simulink model "playback_data_4"  (R2015a)
settings: Solver=FixedStepDiscrete  SolverMode=SingleTasking  StartTime=0  StopTime=time_recorded(end)  FixedStep=sample_time  RelTol=1e-3
undefined symbols (not defined in the file): A1_notch_f1, A2_notch_f1, A_kalman_transverse, A_kalman_vertical, A_lpf_dtau, A_lpf_fourbar_angles, A_lpf_imu, A_lpf_lateral_angle, A_lpf_leg_spring, B1_lpf_dtau, B1_lpf_fourbar_angles, B1_lpf_imu, B1_lpf_lateral_angle, B1_lpf_leg_spring, B1_notch_f1, B2_lpf_dtau, B2_lpf_fourbar_angles, B2_lpf_imu, B2_lpf_lateral_angle, B2_lpf_leg_spring, B2_notch_f1, B_dx_versus_x0, B_kalman_transverse, B_kalman_vertical, backwards_K_front_of_t_row1, backwards_K_front_of_t_row2, backwards_K_sag_of_t, backwards_P_front_of_t, backwards_P_sag_of_t, C_kalman_transverse, C_kalman_vertical, com_leg_motor, com_torso, contact_threshold, control_start_time, d_ankle_to_foot, d_vertical_com, desired_com_forward_velocity, desired_com_lateral_velocity, desired_initial_leg_roll_left, desired_initial_leg_roll_right, desired_lateral_symmetry_angle, desired_standing_torso_pitch, desired_standing_torso_roll, desired_standing_z, desired_torso_pitch, desired_torso_roll, Discrete, fcut_contact, forward_dx_of_dxstar, forward_x_of_dxstar, g, gain_nodes_sea_torque, HIP_MTR_MAX_CONT_TORQUE, HIP_MTR_MAX_TORQUE, i_leg_motor, i_robot, i_torso, initial_dx_estimate, initial_dy_estimate ... (+75)
libraries: simulink x12, ctrlSharedLib x3
(part 2 of 5)

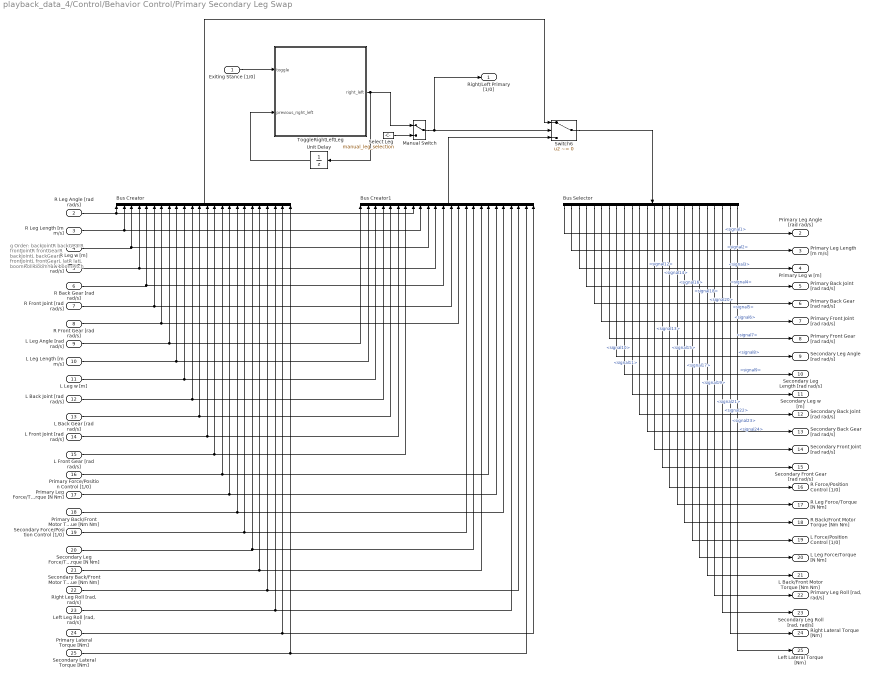
== system playback_data_4/Control/Behavior Control/Primary Secondary Leg Swap ==
  note: q Order:
      |
      | backJointR
      | backGearR
      | frontJointR
      | frontGearR
      |
      | backJointL
      | backGearL
      | frontJointL
      | frontGearL
      |
      | latR
      | latL
      |
      | boomRoll
      | boomYaw
      | boomPitch
  Exiting Stance [1/0] : Inport
  R Leg Angle [rad rad/s] : Inport  Port=2
  R Leg Length [m m/s] : Inport  Port=3
  R Leg w [m] : Inport  Port=4
  R Back Joint [rad rad/s] : Inport  Port=5
  R Back Gear [rad rad/s] : Inport  Port=6
  R Front Joint [rad rad/s] : Inport  Port=7
  R Front Gear [rad rad/s] : Inport  Port=8
  L Leg Angle [rad rad/s] : Inport  Port=9
  L Leg Length [m m/s] : Inport  Port=10
  L Leg w [m] : Inport  Port=11
  L Back Joint [rad rad/s] : Inport  Port=12
  L Back Gear [rad rad/s] : Inport  Port=13
  L Front Joint [rad rad/s] : Inport  Port=14
  L Front Gear [rad rad/s] : Inport  Port=15
  Primary Force/Position Control [1/0] : Inport  Port=16
  Primary Leg Force/Torque [N Nm] : Inport  Port=17
  Primary Back/Front Motor Torque [Nm Nm] : Inport  Port=18
  Secondary Force/Position Control [1/0] : Inport  Port=19
  Secondary Leg Force/Torque [N Nm] : Inport  Port=20
  Secondary Back/Front Motor Torque [Nm Nm] : Inport  Port=21
  "Right Leg Roll [rad, rad/s]" : Inport  Port=22
  "Left Leg Roll [rad, rad/s]" : Inport  Port=23
  Primary Lateral Torque [Nm] : Inport  Port=24
  Secondary Lateral Torque [Nm] : Inport  Port=25
  Bus Creator : BusCreator  Inputs=24
  Bus Creator1 : BusCreator  Inputs=24
  Bus Selector : BusSelector  OutputSignals=signal1,signal2,signal3,signal4,signal5,signal6,signal7,signal8,signal9,signal10,signal11,signal12,signal13,signal14,signal15,signal16,signal17,signal18,signal19,signal20,signal21,signal22,signal23,signal24
  Manual Switch : ManualSwitch
  Select Leg : Constant  Value=manual_leg_selection  OutDataTypeStr=boolean
  Switch6 : Switch  Criteria=u2 ~= 0  OutDataTypeStr=Inherit: Inherit via back propagation  ZeroCross=off
  ToggleRightLeftLeg : MATLAB Function  TreatAsAtomicUnit=on
      settings: MinAlgLoopOccurrences=on
  Unit Delay : UnitDelay  InitialCondition=manual_leg_selection  SampleTime=sample_time
  Right/Left Primary [1/0] : Outport
  Primary Leg Angle [rad rad/s] : Outport  Port=2
  Primary Leg Length [m m/s] : Outport  Port=3
  Primary Leg w [m] : Outport  Port=4
  Primary Back Joint [rad rad/s] : Outport  Port=5
  Primary Back Gear [rad rad/s] : Outport  Port=6
  Primary Front Joint [rad rad/s] : Outport  Port=7
  Primary Front Gear [rad rad/s] : Outport  Port=8
  Secondary Leg Angle [rad rad/s] : Outport  Port=9
  Secondary Leg Length [rad rad/s] : Outport  Port=10
  Secondary Leg w [m] : Outport  Port=11
  Secondary Back Joint [rad rad/s] : Outport  Port=12
  Secondary Back Gear [rad rad/s] : Outport  Port=13
  Secondary Front Joint [rad rad/s] : Outport  Port=14
  Secondary Front Gear [rad rad/s] : Outport  Port=15
  R Force/Position Control [1/0] : Outport  Port=16
  R Leg Force/Torque [N Nm] : Outport  Port=17
  R Back/Front Motor Torque [Nm Nm] : Outport  Port=18
  L Force/Position Control [1/0] : Outport  Port=19
  L Leg Force/Torque [N Nm] : Outport  Port=20
  L Back/Front Motor Torque [Nm Nm] : Outport  Port=21
  "Primary Leg Roll [rad, rad/s]" : Outport  Port=22
  "Secondary Leg Roll [rad, rad/s]" : Outport  Port=23
  Right Lateral Torque [Nm] : Outport  Port=24
  Left Lateral Torque [Nm] : Outport  Port=25
  wires:
  Bus Selector/24 -> Left Lateral Torque [Nm]/1  "<signal24>"
  Bus Selector/23 -> Right Lateral Torque [Nm]/1  "<signal23>"
  Secondary Lateral Torque [Nm]/1 -> Bus Creator/24, Bus Creator1/23
  Primary Lateral Torque [Nm]/1 -> Bus Creator/23, Bus Creator1/24
  Bus Selector/22 -> "Secondary Leg Roll [rad, rad/s]"/1  "<signal22>"
  Bus Selector/21 -> "Primary Leg Roll [rad, rad/s]"/1  "<signal21>"
  "Left Leg Roll [rad, rad/s]"/1 -> Bus Creator/22, Bus Creator1/21
  "Right Leg Roll [rad, rad/s]"/1 -> Bus Creator/21, Bus Creator1/22
  Bus Selector/20 -> L Back/Front Motor Torque [Nm Nm]/1  "<signal20>"
  Bus Selector/19 -> L Leg Force/Torque [N Nm]/1  "<signal19>"
  Bus Selector/18 -> L Force/Position Control [1/0]/1  "<signal18>"
  Bus Selector/17 -> R Back/Front Motor Torque [Nm Nm]/1  "<signal17>"
  Bus Selector/16 -> R Leg Force/Torque [N Nm]/1  "<signal16>"
  Bus Selector/15 -> R Force/Position Control [1/0]/1  "<signal15>"
  Bus Selector/14 -> Secondary Front Gear [rad rad/s]/1  "<signal14>"
  Bus Selector/13 -> Secondary Front Joint [rad rad/s]/1  "<signal13>"
  Bus Selector/12 -> Secondary Back Gear [rad rad/s]/1  "<signal12>"
  Bus Selector/11 -> Secondary Back Joint [rad rad/s]/1  "<signal11>"
  Bus Selector/10 -> Secondary Leg w [m]/1  "<signal10>"
  Bus Selector/9 -> Secondary Leg Length [rad rad/s]/1  "<signal9>"
  Bus Selector/8 -> Secondary Leg Angle [rad rad/s]/1  "<signal8>"
  Bus Selector/7 -> Primary Front Gear [rad rad/s]/1  "<signal7>"
  Bus Selector/6 -> Primary Front Joint [rad rad/s]/1  "<signal6>"
  Bus Selector/5 -> Primary Back Gear [rad rad/s]/1  "<signal5>"
  Bus Selector/4 -> Primary Back Joint [rad rad/s]/1  "<signal4>"
  Bus Selector/3 -> Primary Leg w [m]/1  "<signal3>"
  Bus Selector/2 -> Primary Leg Length [m m/s]/1  "<signal2>"
  Bus Selector/1 -> Primary Leg Angle [rad rad/s]/1  "<signal1>"
  Switch6/1 -> Bus Selector/1
  Secondary Back/Front Motor Torque [Nm Nm]/1 -> Bus Creator/20, Bus Creator1/17
  Secondary Leg Force/Torque [N Nm]/1 -> Bus Creator/19, Bus Creator1/16
  Secondary Force/Position Control [1/0]/1 -> Bus Creator/18, Bus Creator1/15
  Primary Back/Front Motor Torque [Nm Nm]/1 -> Bus Creator/17, Bus Creator1/20
  Primary Leg Force/Torque [N Nm]/1 -> Bus Creator/16, Bus Creator1/19
  Primary Force/Position Control [1/0]/1 -> Bus Creator/15, Bus Creator1/18
  L Front Gear [rad rad/s]/1 -> Bus Creator/14, Bus Creator1/7
  L Front Joint [rad rad/s]/1 -> Bus Creator1/6, Bus Creator/13
  L Back Gear [rad rad/s]/1 -> Bus Creator/12, Bus Creator1/5
  L Back Joint [rad rad/s]/1 -> Bus Creator/11, Bus Creator1/4
  L Leg w [m]/1 -> Bus Creator/10, Bus Creator1/3
  L Leg Length [m m/s]/1 -> Bus Creator/9, Bus Creator1/2
  L Leg Angle [rad rad/s]/1 -> Bus Creator/8, Bus Creator1/1
  R Front Gear [rad rad/s]/1 -> Bus Creator/7, Bus Creator1/14
  R Front Joint [rad rad/s]/1 -> Bus Creator/6, Bus Creator1/13
  R Back Gear [rad rad/s]/1 -> Bus Creator/5, Bus Creator1/12
  R Back Joint [rad rad/s]/1 -> Bus Creator/4, Bus Creator1/11
  Bus Creator1/1 -> Switch6/3
  Bus Creator/1 -> Switch6/1
  R Leg Length [m m/s]/1 -> Bus Creator/2, Bus Creator1/9
  R Leg Angle [rad rad/s]/1 -> Bus Creator/1, Bus Creator1/8
  R Leg w [m]/1 -> Bus Creator/3, Bus Creator1/10
  Select Leg/1 -> Manual Switch/2
  Manual Switch/1 -> Switch6/2, Right/Left Primary [1/0]/1
  ToggleRightLeftLeg/1(right_left) -> Manual Switch/1, Unit Delay/1
  Exiting Stance [1/0]/1 -> ToggleRightLeftLeg/1(toggle)
  Unit Delay/1 -> ToggleRightLeftLeg/2(previous_right_left)

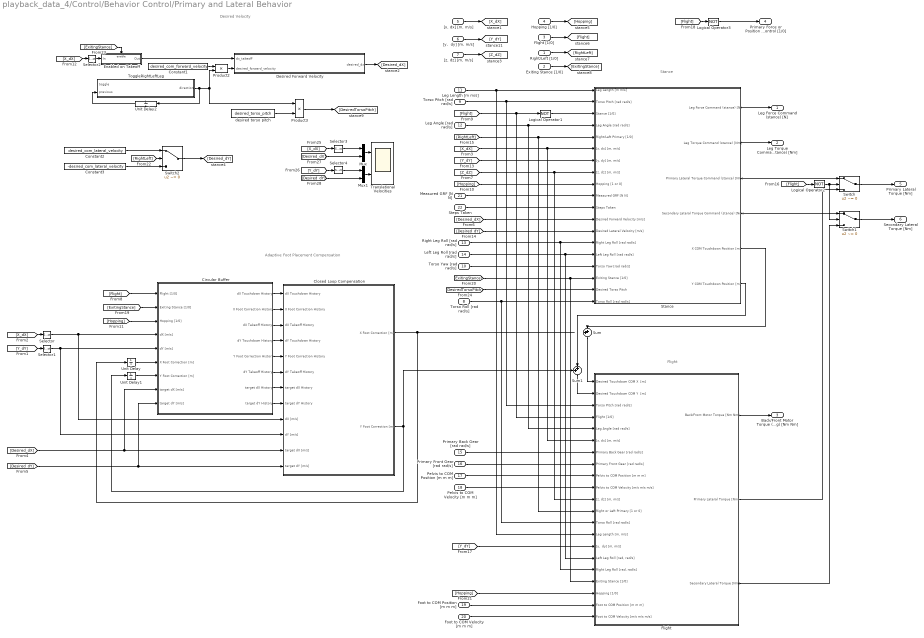
== system playback_data_4/Control/Behavior Control/Primary and Lateral Behavior ==
  note: Desired Velocity
  note: Adaptive Foot Placement Compensation
  note: Flight
  note: Stance
  Right/Left [1/0] : Inport
  Exiting Stance [1/0] : Inport  Port=2
  Flight [1/0] : Inport  Port=3
  Hopping [1/0] : Inport  Port=4
  "[x, dx] [m, m/s]" : Inport  Port=5
  "[y,  dy] [m, m/s]" : Inport  Port=6
  "[z, dz] [m, m/s]" : Inport  Port=7
  Torso Roll [rad rad/s] : Inport  Port=8
  Torso Pitch [rad rad/s] : Inport  Port=9
  Torso Yaw [rad rad/s] : Inport  Port=10
  Leg Length [m m/s] : Inport  Port=11
  Leg Angle [rad rad/s] : Inport  Port=12
  Right Leg Roll [rad rad/s] : Inport  Port=13
  Left Leg Roll [rad rad/s] : Inport  Port=14
  Primary Back Gear [rad rad/s] : Inport  Port=15
  Primary Front Gear [rad rad/s] : Inport  Port=16
  Pelvis to COM Position [m m m] : Inport  Port=17
  Pelvis to COM Velocity [m m m] : Inport  Port=18
  Foot to COM Position [m m m] : Inport  Port=19
  Foot to COM Velocity [m m m] : Inport  Port=20
  Measured GRF [N N] : Inport  Port=21
  Steps Taken : Inport  Port=22
  Circular Buffer : Subsystem
  Closed Loop Compensation : Subsystem
  Constant1 : Constant  Value=desired_com_forward_velocity
  Constant2 : Constant  Value=desired_com_lateral_velocity
  Constant3 : Constant  Value=-desired_com_lateral_velocity
  Desired Forward Velocity : MATLAB Function  TreatAsAtomicUnit=on
  Enabled on Takeoff : Subsystem  TreatAsAtomicUnit=on
  Flight : Subsystem
  Logical Operator1 : Logic  Operator=NOT  AllPortsSameDT=off  OutDataTypeStr=boolean
  Logical Operator2 : Logic  Operator=NOT  AllPortsSameDT=off  OutDataTypeStr=boolean
  Logical Operator3 : Logic  Operator=NOT  AllPortsSameDT=off  OutDataTypeStr=boolean
  Mux : Mux  Inputs=2
  Mux1 : Mux  Inputs=2
  Product2 : Product
  Product3 : Product
  Selector{,1..4} (5 alike) : Selector  InputPortWidth=2  Indices=[2]
  Stance : Subsystem
  Sum : Sum  Inputs=++|
  Sum1 : Sum  Inputs=++|
  Switch : Switch  Criteria=u2 ~= 0
  Switch1 : Switch  Criteria=u2 ~= 0
  Switch2 : Switch  Criteria=u2 ~= 0
  ToggleRightLeftLeg : MATLAB Function  TreatAsAtomicUnit=on
      settings: MinAlgLoopOccurrences=on
  Translational Velocities : Scope  NumInputPorts=2
      settings: YMin=-1000~-5  YMax=1000~5  SaveName=ScopeData2  SampleInput=on
  Unit Delay : UnitDelay  SampleTime=-1
  Unit Delay1 : UnitDelay  SampleTime=-1
  Unit Delay2 : UnitDelay  InitialCondition=1  SampleTime=sample_time
  desired torso pitch : Constant  Value=desired_torso_pitch
  Leg Force Command (stance) [N] : Outport
  Leg Torque Command (stance) [Nm] : Outport  Port=2
  Back/Front Motor Torque (swing) [Nm Nm] : Outport  Port=3
  Primary Force or Position Control [1/0] : Outport  Port=4  OutDataTypeStr=boolean
  Primary Lateral Torque [Nm] : Outport  Port=5
  Secondary Lateral Torque [Nm] : Outport  Port=6
  wires:
  [Desired_dX] -> Mux/2
  [Desired_dY] -> Mux1/2
  Mux1/1 -> Translational Velocities/2
  Mux/1 -> Translational Velocities/1
  Selector4/1 -> Mux1/1
  [Y_dY] -> Selector4/1
  Selector3/1 -> Mux/1
  [X_dX] -> Selector3/1
  Foot to COM Velocity [m m m]/1 -> Flight/21(Foot to COM Velocity [m/s m/s m/s])
  Foot to COM Position [m m m]/1 -> Flight/20(Foot to COM Position [m m m])
  [DesiredTorsoPitch] -> Stance/18(Desired Torso Pitch)
  Product3/1 -> [DesiredTorsoPitch]
  desired torso pitch/1 -> Product3/2
  Constant1/1 -> Product2/1
  Unit Delay2/1 -> ToggleRightLeftLeg/2(previous)
  ToggleRightLeftLeg/1(direction) -> Unit Delay2/1, Product3/1, Product2/2
  Product2/1 -> Desired Forward Velocity/2(desired_forward_velocity)
  Desired Forward Velocity/1(desired_dx) -> [Desired_dX]
  Selector2/1 -> Enabled on Takeoff/1(In)
  [ExitingStance] -> Enabled on Takeoff/Enable
  Constant3/1 -> Switch2/3
  Constant2/1 -> Switch2/1
  [RightLeft] -> Switch2/2
  Enabled on Takeoff/1(Out) -> Desired Forward Velocity/1(dx_takeoff)
  Switch2/1 -> [Desired_dY]
  [X_dX] -> Selector2/1
  [Hopping] -> Flight/19(Hopping [1/0])
  [ExitingStance] -> Flight/18(Exiting Stance [1/0]), Stance/17(Exiting Stance [1/0])
  Exiting Stance [1/0]/1 -> [ExitingStance]
  [ExitingStance] -> Circular Buffer/2(Exiting Stance [1/0])
  [Hopping] -> Circular Buffer/3(Hopping [1/0])
  Torso Yaw [rad rad/s]/1 -> Stance/16(Torso Yaw [rad rad/s])
  Logical Operator3/1 -> Primary Force or Position Control [1/0]/1
  [Flight] -> Logical Operator3/1
  Switch1/1 -> Secondary Lateral Torque [Nm]/1
  Switch/1 -> Primary Lateral Torque [Nm]/1
  [Flight] -> Logical Operator2/1
  Flight/3(Secondary Lateral Torque [Nm]) -> Switch1/3
  Stance/4(Secondary Lateral Torque Command (stance) [Nm]) -> Switch1/1
  Flight/2(Primary Lateral Torque [Nm]) -> Switch/3
  Stance/3(Primary Lateral Torque Command (stance) [Nm]) -> Switch/1
  Logical Operator2/1 -> Switch/2, Switch1/2
  Right/Left [1/0]/1 -> [RightLeft]
  [Desired_dY] -> Stance/13(Desired Lateral Velocity [m/s])
  [Y_dY] -> Stance/7("[y, dy] [m, m/s]")
  Left Leg Roll [rad rad/s]/1 -> Flight/16("Left Leg Roll [rad, rad/s]"), Stance/15(Left Leg Roll [rad rad/s])
  Right Leg Roll [rad rad/s]/1 -> Flight/17("Right Leg Roll [rad, rad/s]"), Stance/14(Right Leg Roll [rad rad/s])
  Sum1/1 -> Flight/2(Desired Touchdown COM Y  [m])
  Stance/6(Y COM Touchdown Position [m]) -> Sum1/2
  Hopping [1/0]/1 -> [Hopping]
  [Flight] -> Logical Operator1/1, Flight/4(Flight [1/0])
  Flight [1/0]/1 -> [Flight]
  [Desired_dX] -> Stance/12(Desired Forward Velocity [m/s])
  [Y_dY] -> Selector1/1
  [X_dX] -> Selector/1
  "[y,  dy] [m, m/s]"/1 -> [Y_dY]
  "[z, dz] [m, m/s]"/1 -> [Z_dZ]
  "[x, dx] [m, m/s]"/1 -> [X_dX]
  Closed Loop Compensation/2(Y Foot Correction [m]) -> Sum1/1, Unit Delay1/1
  Unit Delay/1 -> Circular Buffer/6(X Foot Correction [m])
  Unit Delay1/1 -> Circular Buffer/7(Y Foot Correction [m])
  Selector/1 -> Circular Buffer/4(dX [m/s]), Closed Loop Compensation/9(dX [m/s])
  Selector1/1 -> Circular Buffer/5(dY [m/s]), Closed Loop Compensation/10(dY [m/s])
  Closed Loop Compensation/1(X Foot Correction [m]) -> Unit Delay/1
  Sum/1 -> Flight/1(Desired Touchdown COM X  [m])
  Stance/5(X COM Touchdown Position [m]) -> Sum/2
  [Desired_dY] -> Closed Loop Compensation/12("target dY [m/s] "), Circular Buffer/9(target dY [m/s])
  [Desired_dX] -> Closed Loop Compensation/11(target dX [m/s]), Circular Buffer/8(target dX [m/s])
  Circular Buffer/7(target dX History) -> Closed Loop Compensation/7(target dX History)
  Circular Buffer/8(target dY History) -> Closed Loop Compensation/8(target dY History)
  Circular Buffer/6(dY Takeoff History) -> Closed Loop Compensation/6(dY Takeoff History)
  Circular Buffer/5(Y Foot Correction History) -> Closed Loop Compensation/5(Y Foot Correction History)
  Circular Buffer/4("dY Touchdown History ") -> Closed Loop Compensation/4(dY Touchdown History)
  Circular Buffer/3(dX Takeoff History) -> Closed Loop Compensation/3(dX Takeoff History)
  Circular Buffer/2(X Foot Correction History) -> Closed Loop Compensation/2(X Foot Correction History)
  Circular Buffer/1("dX Touchdown History ") -> Closed Loop Compensation/1(dX Touchdown History)
  [Y_dY] -> Flight/15("[y,  dy] [m, m/s]")
  Steps Taken/1 -> Stance/11(Steps Taken)
  Measured GRF [N N]/1 -> Stance/10(Measured GRF [N N])
  Torso Roll [rad rad/s]/1 -> Flight/13(Torso Roll [rad rad/s]), Stance/19(Torso Roll [rad rad/s])
  Pelvis to COM Velocity [m m m]/1 -> Flight/10(Pelvis to COM Velocity [m/s m/s m/s])
  [Z_dZ] -> Flight/11("[z, dz] [m, m/s]"), Stance/8("[z, dz] [m, m/s]")
  Pelvis to COM Position [m m m]/1 -> Flight/9(Pelvis to COM Position [m m m])
  [Flight] -> Circular Buffer/1(Flight [1/0])
  Logical Operator1/1 -> Stance/3(Stance [1/0])
  Flight/1(Back/Front Motor Torque [Nm Nm]) -> Back/Front Motor Torque (swing) [Nm Nm]/1
  Leg Angle [rad rad/s]/1 -> Flight/5(Leg Angle [rad rad/s]), Stance/4(Leg Angle [rad rad/s])
  Primary Front Gear [rad rad/s]/1 -> Flight/8(Primary Front Gear [rad rad/s])
  Primary Back Gear [rad rad/s]/1 -> Flight/7(Primary Back Gear [rad rad/s])
  [RightLeft] -> Flight/12(Right or Left Primary [1 or 0]), Stance/5(Right/Left Primary [1/0])
  [X_dX] -> Flight/6("[x, dx] [m, m/s]"), Stance/6("[x, dx] [m, m/s]")
  [Hopping] -> Stance/9(Hopping [1 or 0])
  Torso Pitch [rad rad/s]/1 -> Flight/3(Torso Pitch [rad rad/s]), Stance/2(Torso Pitch [rad rad/s])
  Stance/2(Leg Torque Command (stance) [Nm]) -> Leg Torque Command (stance) [Nm]/1
  Stance/1(Leg Force Command (stance) [N]) -> Leg Force Command (stance) [N]/1
  Leg Length [m m/s]/1 -> Flight/14("Leg Length [m, m/s]"), Stance/1(Leg Length [m m/s])

== system playback_data_4/Control/Behavior Control/R Leg Calculator ==
  Front [rad rad/s] : Inport
  Back [rad rad/s] : Inport  Port=2
  Constant : Constant  Value=d_ankle_to_foot-0.01
  Demux1 : Demux  Outputs=2
  Gain1 : Gain  Gain=2*l_seg
  Gain2 : Gain  Gain=l_seg
  Gain3 : Gain  Gain=-1
  Gain4 : Gain  Gain=0.5
  Gain5 : Gain  Gain=0.5
  Gain6 : Gain  Gain=2
  Mux1 : Mux  Inputs=2
  Product : Product  RndMeth=Zero
  Sum : Sum  Inputs=++|
  Sum4 : Sum  Inputs=+|+
  Sum5 : Sum  Inputs=+|-
  Trigonometric Function : Trigonometry  Operator=cos
  Trigonometric Function1 : Trigonometry
  "Leg Length [m m/s] " : Outport
  Leg Angle [rad rad/s] : Outport  Port=2
  Leg Splay [rad rad/s] : Outport  Port=3
  w [m] : Outport  Port=4
  wires:
  Gain5/1 -> Leg Angle [rad rad/s]/1
  Sum4/1 -> Gain5/1
  Mux1/1 -> "Leg Length [m m/s] "/1
  Sum5/1 -> Demux1/1, Leg Splay [rad rad/s]/1
  Gain2/1 -> Gain6/1, Product/1
  Demux1/1 -> Gain4/1
  Gain3/1 -> Product/2
  Demux1/2 -> Gain3/1
  Back [rad rad/s]/1 -> Sum5/1, Sum4/1
  Front [rad rad/s]/1 -> Sum4/2, Sum5/2
  Product/1 -> Mux1/2
  Trigonometric Function1/1 -> Gain2/1
  Gain1/1 -> Sum/2
  Trigonometric Function/1 -> Gain1/1
  Gain4/1 -> Trigonometric Function/1, Trigonometric Function1/1
  Gain6/1 -> w [m]/1
  Sum/1 -> Mux1/1
  Constant/1 -> Sum/1

== system playback_data_4/Control/Behavior Control/Secondary Leg Behavior ==
  note: Convert to
      | four-bar angles
  note: Position control the
      | individual four bar segments
  note: Mirror the primary
      | leg motion
  Secondary Back Gear [rad rad/s] : Inport
  Secondary Front Gear [rad rad/s] : Inport  Port=2
  Torso Pitch [rad rad/s] : Inport  Port=3
  Right/Left Secondary [1/0] : Inport  Port=4
  Primary Leg Angle [rad rad/s] : Inport  Port=5
  Primary Leg Length [m m/s] : Inport  Port=6
  Avoid Hitting Mechanical Limits : MATLAB Function  TreatAsAtomicUnit=on
  Back/Front Motor PD : Subsystem
  Constant4 : Constant  Value=0
  Constant5 : Constant  Value=0  OutDataTypeStr=boolean
  Demux{1..3,5} (4 alike) : Demux  Outputs=2
  Demux6 : Demux  Outputs=6
  Fcn2 : Fcn  Expr=2*pi-u(1)
  Mirrored Leg Length Target : MATLAB Function  TreatAsAtomicUnit=on
  Mux{1..4,7,11} (6 alike) : Mux  Inputs=2
  Mux5 : Mux  Inputs=3
  Mux6 : Mux  Inputs=3
  Sum1 : Sum  Inputs=++|
  Virtual Leg to Four Bar : MATLAB Function  TreatAsAtomicUnit=on
  k_virtual6 : Gain  Gain=-1
  two_pole_filter : DiscreteTransferFcn  Numerator=[A_lpf_leg_spring 0 0]  Denominator=[1 B1_lpf_leg_spring B2_lpf_leg_spring]  SampleTime=sample_time
  Secondary Back/Front Motor Torque [Nm Nm] : Outport
  Secondary Force or Position Control [1/0] : Outport  Port=2
  wires:
  Back/Front Motor PD/1(Commanded Torque [Nm] [back front]) -> Secondary Back/Front Motor Torque [Nm Nm]/1
  Primary Leg Length [m m/s]/1 -> Demux1/1
  Demux1/2 -> Mirrored Leg Length Target/2(primary_dl_leg)
  Demux1/1 -> Mirrored Leg Length Target/1(primary_l_leg)
  Sum1/1 -> Demux5/1
  two_pole_filter/1 -> Sum1/2
  Mux3/1 -> Back/Front Motor PD/3(Desired Acceleration [rad/s^2] [back front])
  Mux2/1 -> Back/Front Motor PD/2(Desired Velocity [rad/s] [back front])
  Avoid Hitting Mechanical Limits/6(ddfront_cmd) -> Mux3/2
  Avoid Hitting Mechanical Limits/5(ddback_cmd) -> Mux3/1
  Avoid Hitting Mechanical Limits/4(dfront_cmd) -> Mux2/2
  Avoid Hitting Mechanical Limits/3(dback_cmd) -> Mux2/1
  Secondary Back Gear [rad rad/s]/1 -> Demux3/1
  Secondary Front Gear [rad rad/s]/1 -> Demux2/1
  Demux2/1 -> Mux4/2
  Avoid Hitting Mechanical Limits/1(back_cmd) -> Mux1/1
  Avoid Hitting Mechanical Limits/2(front_cmd) -> Mux1/2
  Demux3/1 -> Mux4/1
  Demux3/2 -> Mux11/1
  Right/Left Secondary [1/0]/1 -> Back/Front Motor PD/6(Right/Left Leg [1/0])
  Mux1/1 -> Back/Front Motor PD/1(Desired Position [rad] [back front])
  Mux4/1 -> Back/Front Motor PD/4(Measured Position [rad] [back front])
  Demux2/2 -> Mux11/2
  Mux11/1 -> Back/Front Motor PD/5(Measured Velocity [rad/s] [back front])
  Demux6/6 -> Virtual Leg to Four Bar/6(ddphi)
  Demux6/5 -> Virtual Leg to Four Bar/5(dphi)
  Demux6/4 -> Virtual Leg to Four Bar/4(phi)
  Demux6/3 -> Virtual Leg to Four Bar/3(ddl_leg)
  Demux6/2 -> Virtual Leg to Four Bar/2(dl_leg)
  Demux6/1 -> Virtual Leg to Four Bar/1(l_leg)
  Virtual Leg to Four Bar/6(ddfront) -> Avoid Hitting Mechanical Limits/6(ddfront_desired)
  Virtual Leg to Four Bar/5(dfront) -> Avoid Hitting Mechanical Limits/5(dfront_desired)
  Virtual Leg to Four Bar/4(front) -> Avoid Hitting Mechanical Limits/4(front_desired)
  Virtual Leg to Four Bar/3(ddback) -> Avoid Hitting Mechanical Limits/3(ddback_desired)
  Virtual Leg to Four Bar/2(dback) -> Avoid Hitting Mechanical Limits/2(dback_desired)
  Virtual Leg to Four Bar/1(back) -> Avoid Hitting Mechanical Limits/1(back_desired)
  Mux6/1 -> Mux7/2
  Mux5/1 -> Mux7/1
  Torso Pitch [rad rad/s]/1 -> Sum1/1
  Mux7/1 -> Demux6/1
  Fcn2/1 -> Mux6/1
  k_virtual6/1 -> Mux6/2
  Constant4/1 -> Mux6/3
  Mirrored Leg Length Target/1(l_leg) -> Mux5/1
  Mirrored Leg Length Target/3(ddl_leg) -> Mux5/3
  Mirrored Leg Length Target/2(dl_leg) -> Mux5/2
  Primary Leg Angle [rad rad/s]/1 -> two_pole_filter/1
  Demux5/1 -> Fcn2/1
  Demux5/2 -> k_virtual6/1
  Constant5/1 -> Secondary Force or Position Control [1/0]/1

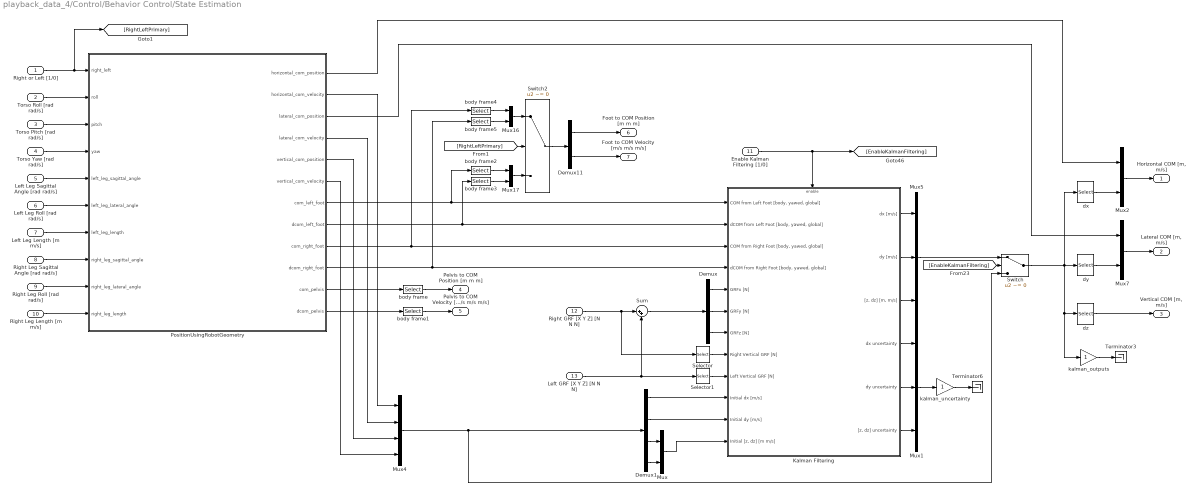
== system playback_data_4/Control/Behavior Control/State Estimation ==
  Right or Left [1/0] : Inport
  Torso Roll [rad rad/s] : Inport  Port=2
  Torso Pitch [rad rad/s] : Inport  Port=3
  Torso Yaw [rad rad/s] : Inport  Port=4
  Left Leg Sagittal Angle [rad rad/s] : Inport  Port=5
  Left Leg Roll [rad rad/s] : Inport  Port=6
  Left Leg Length [m m/s] : Inport  Port=7
  Right Leg Sagittal Angle [rad rad/s] : Inport  Port=8
  Right Leg Roll [rad rad/s] : Inport  Port=9
  Right Leg Length [m m/s] : Inport  Port=10
  Enable Kalman Filtering [1/0] : Inport  Port=11
  Right GRF [X Y Z] [N N N] : Inport  Port=12
  Left GRF [X Y Z] [N N N] : Inport  Port=13
  Demux : Demux  Outputs=3
  Demux1 : Demux
  Demux11 : Demux  Outputs=2
  Kalman Filtering : Subsystem
  Mux{,2,7,16..17} (5 alike) : Mux  Inputs=2
  Mux1 : Mux  Inputs=3
  Mux4 : Mux
  Mux5 : Mux  Inputs=3
  PositionUsingRobotGeometry : MATLAB Function  TreatAsAtomicUnit=on
  Selector : Selector  InputPortWidth=3  Indices=[3]
  Selector1 : Selector  InputPortWidth=3  Indices=[3]
  Sum : Sum  Inputs=|++
  Switch : Switch  Criteria=u2 ~= 0
  Switch2 : Switch  Criteria=u2 ~= 0
  Terminator3 : Terminator
  Terminator6 : Terminator
  body frame : Selector  InputPortWidth=9  Indices=[1 2 3]
  body frame1 : Selector  InputPortWidth=9  Indices=[1 2 3]
  body frame{2..5} (4 alike) : Selector  InputPortWidth=9  Indices=[4 5 6]
  dx : Selector  InputPortWidth=4  Indices=[1]
  dy : Selector  InputPortWidth=4  Indices=[2]
  dz : Selector  InputPortWidth=4  Indices=[3 4]
  kalman_outputs : Gain
  kalman_uncertainty : Gain
  "Horizontal COM [m, m/s]" : Outport
  "Lateral COM [m, m/s]" : Outport  Port=2
  "Vertical COM [m, m/s]" : Outport  Port=3
  Pelvis to COM Position [m m m] : Outport  Port=4
  Pelvis to COM Velocity [m/s m/s m/s] : Outport  Port=5
  Foot to COM Position [m m m] : Outport  Port=6
  Foot to COM Velocity [m/s m/s m/s] : Outport  Port=7
  wires:
  body frame4/1 -> Mux16/1
  body frame5/1 -> Mux16/2
  body frame3/1 -> Mux17/2
  body frame2/1 -> Mux17/1
  Demux11/1 -> Foot to COM Position [m m m]/1
  Demux11/2 -> Foot to COM Velocity [m/s m/s m/s]/1
  Switch2/1 -> Demux11/1
  Mux16/1 -> Switch2/1
  Mux17/1 -> Switch2/3
  [RightLeftPrimary] -> Switch2/2
  Demux1/1 -> Kalman Filtering/10(Initial dx [m/s])
  Demux1/2 -> Kalman Filtering/11(Initial dy [m/s])
  Mux/1 -> Kalman Filtering/12("Initial [z, dz] [m m/s]")
  Demux1/4 -> Mux/2
  Demux1/3 -> Mux/1
  Mux4/1 -> Switch/3, Demux1/1
  [EnableKalmanFiltering] -> Switch/2
  dy/1 -> Mux7/2
  Mux1/1 -> kalman_uncertainty/1
  Kalman Filtering/6("[z, dz] uncertainty") -> Mux1/3
  Kalman Filtering/4(dx uncertainty) -> Mux1/1
  Kalman Filtering/5(dy uncertainty) -> Mux1/2
  Kalman Filtering/2(dy [m/s]) -> Mux5/2
  Kalman Filtering/3("[z, dz] [m, m/s]") -> Mux5/3
  Kalman Filtering/1(dx [m/s]) -> Mux5/1
  Demux/2 -> Kalman Filtering/6(GRFy [N])
  Demux/3 -> Kalman Filtering/7(GRFz [N])
  Mux7/1 -> "Lateral COM [m, m/s]"/1
  Switch/1 -> kalman_outputs/1, dz/1, dy/1, dx/1
  dz/1 -> "Vertical COM [m, m/s]"/1
  PositionUsingRobotGeometry/2(horizontal_com_velocity) -> Mux4/1
  PositionUsingRobotGeometry/3(lateral_com_position) -> Mux7/1
  PositionUsingRobotGeometry/4(lateral_com_velocity) -> Mux4/2
  PositionUsingRobotGeometry/5(vertical_com_position) -> Mux4/3
  PositionUsingRobotGeometry/6(vertical_com_velocity) -> Mux4/4
  body frame1/1 -> Pelvis to COM Velocity [m/s m/s m/s]/1
  body frame/1 -> Pelvis to COM Position [m m m]/1
  Mux2/1 -> "Horizontal COM [m, m/s]"/1
  PositionUsingRobotGeometry/11(com_pelvis) -> body frame/1
  PositionUsingRobotGeometry/12(dcom_pelvis) -> body frame1/1
  kalman_uncertainty/1 -> Terminator6/1
  Demux/1 -> Kalman Filtering/5(GRFx [N])
  kalman_outputs/1 -> Terminator3/1
  Enable Kalman Filtering [1/0]/1 -> Kalman Filtering/Enable, [EnableKalmanFiltering]
  Sum/1 -> Demux/1
  Right GRF [X Y Z] [N N N]/1 -> Sum/1, Selector/1
  Left GRF [X Y Z] [N N N]/1 -> Sum/2, Selector1/1
  Selector1/1 -> Kalman Filtering/9(Left Vertical GRF [N])
  Selector/1 -> Kalman Filtering/8(Right Vertical GRF [N])
  Mux5/1 -> Switch/1
  dx/1 -> Mux2/2
  PositionUsingRobotGeometry/10(dcom_right_foot) -> Kalman Filtering/4("dCOM from Right Foot [body, yawed, global]"), body frame5/1
  PositionUsingRobotGeometry/9(com_right_foot) -> Kalman Filtering/3("COM from Right Foot [body, yawed, global]"), body frame4/1
  PositionUsingRobotGeometry/8(dcom_left_foot) -> Kalman Filtering/2("dCOM from Left Foot [body, yawed, global]"), body frame3/1
  PositionUsingRobotGeometry/7(com_left_foot) -> Kalman Filtering/1("COM from Left Foot [body, yawed, global]"), body frame2/1
  Torso Pitch [rad rad/s]/1 -> PositionUsingRobotGeometry/3(pitch)
  Torso Yaw [rad rad/s]/1 -> PositionUsingRobotGeometry/4(yaw)
  Torso Roll [rad rad/s]/1 -> PositionUsingRobotGeometry/2(roll)
  Right or Left [1/0]/1 -> PositionUsingRobotGeometry/1(right_left), [RightLeftPrimary]
  Right Leg Length [m m/s]/1 -> PositionUsingRobotGeometry/10(right_leg_length)
  Right Leg Roll [rad rad/s]/1 -> PositionUsingRobotGeometry/9(right_leg_lateral_angle)
  Right Leg Sagittal Angle [rad rad/s]/1 -> PositionUsingRobotGeometry/8(right_leg_sagittal_angle)
  Left Leg Length [m m/s]/1 -> PositionUsingRobotGeometry/7(left_leg_length)
  Left Leg Roll [rad rad/s]/1 -> PositionUsingRobotGeometry/6(left_leg_lateral_angle)
  Left Leg Sagittal Angle [rad rad/s]/1 -> PositionUsingRobotGeometry/5(left_leg_sagittal_angle)
  PositionUsingRobotGeometry/1(horizontal_com_position) -> Mux2/1

== system playback_data_4/Control/Behavior Control/Torque Distribution Left ==
  Leg Torque [Nm] : Inport
  Leg Force [N] : Inport  Port=2
  w [m] : Inport  Port=3
  Gain : Gain  Gain=0.5
  Gain1 : Gain  Gain=0.5
  Motor Torque Saturation Optimization : MATLAB Function  TreatAsAtomicUnit=on
  Product : Product  RndMeth=Zero
  Sum : Sum  Inputs=|++
  Sum1 : Sum  Inputs=+-|
  Back Torque [Nm] : Outport
  Front Torque [Nm] : Outport  Port=2
  wires:
  Sum1/1 -> Back Torque [Nm]/1
  Leg Torque [Nm]/1 -> Gain/1
  Sum/1 -> Front Torque [Nm]/1
  Motor Torque Saturation Optimization/1(t1) -> Sum/1, Sum1/1
  w [m]/1 -> Product/2
  Motor Torque Saturation Optimization/2(t2) -> Sum1/2, Sum/2
  Leg Force [N]/1 -> Product/1
  Product/1 -> Gain1/1
  Gain1/1 -> Motor Torque Saturation Optimization/2(x2s)
  Gain/1 -> Motor Torque Saturation Optimization/1(x1s)

== system playback_data_4/Control/Behavior Control/Torque Distribution Right ==
  Leg Torque [Nm] : Inport
  Leg Force [N] : Inport  Port=2
  w [m] : Inport  Port=3
  Gain : Gain  Gain=0.5
  Gain1 : Gain  Gain=0.5
  Motor Torque Saturation Optimization : MATLAB Function  TreatAsAtomicUnit=on
  Product : Product  RndMeth=Zero
  Sum : Sum  Inputs=|++
  Sum1 : Sum  Inputs=+-|
  Back Torque [Nm] : Outport
  Front Torque [Nm] : Outport  Port=2
  wires:
  Gain/1 -> Motor Torque Saturation Optimization/1(x1s)
  Gain1/1 -> Motor Torque Saturation Optimization/2(x2s)
  Product/1 -> Gain1/1
  Leg Force [N]/1 -> Product/1
  Motor Torque Saturation Optimization/2(t2) -> Sum/2, Sum1/2
  w [m]/1 -> Product/2
  Motor Torque Saturation Optimization/1(t1) -> Sum1/1, Sum/1
  Sum/1 -> Front Torque [Nm]/1
  Leg Torque [Nm]/1 -> Gain/1
  Sum1/1 -> Back Torque [Nm]/1

== system playback_data_4/Control/Subsystem/Activate SEA Control ==
  SEA Control Signal [Nm] x4 : Inport
  "SEA on/off [1/0] x4 " : Inport  Port=2
  Torque Signal [Nm] x4 : Inport  Port=3
  Demux : Demux
  Demux2 : Demux
  Demux3 : Demux
  Mux6 : Mux
  Switch{,1..3} (4 alike) : Switch  Criteria=u2 ~= 0
  Torque Command [Nm] x4 : Outport
  wires:
  Demux2/2 -> Switch1/3
  Demux2/1 -> Switch/3
  Demux/1 -> Switch/1
  Switch/1 -> Mux6/1
  Switch1/1 -> Mux6/2
  Switch3/1 -> Mux6/4
  Demux3/1 -> Switch/2
  Mux6/1 -> Torque Command [Nm] x4/1
  Demux3/3 -> Switch2/2
  Demux3/2 -> Switch1/2
  Demux/3 -> Switch2/1
  Switch2/1 -> Mux6/3
  Demux/4 -> Switch3/1
  Demux2/4 -> Switch3/3
  Demux3/4 -> Switch3/2
  Demux/2 -> Switch1/1
  Demux2/3 -> Switch2/3
  SEA Control Signal [Nm] x4/1 -> Demux/1
  "SEA on/off [1/0] x4 "/1 -> Demux3/1
  Torque Signal [Nm] x4/1 -> Demux2/1

== system playback_data_4/Control/Subsystem/Antiresonance Compensation ==
  Torque : Inport
  Notch Filter (Flight) : DiscreteTransferFcn  Numerator=[K_notch_f1 K_notch_f1*A1_notch_f1 K_notch_f1*A2_notch_f1]  Denominator=[1 B1_notch_f1 B2_notch_f1]  SampleTime=sample_time
  Filtered Torque : Outport
  wires:
  Torque/1 -> Notch Filter (Flight)/1
  Notch Filter (Flight)/1 -> Filtered Torque/1

== system playback_data_4/Control/Subsystem/Compare SEA Signals ==
  Enabled : Inport
  Measured : Inport  Port=2
  Desired : Inport  Port=3
  Demux : Demux
  Demux1 : Demux
  Demux2 : Demux
  Mux{6..9} (4 alike) : Mux  Inputs=2
  Product{,1..3} (4 alike) : Product
  RB : Outport
  RF : Outport  Port=2
  LB : Outport  Port=3
  LF : Outport  Port=4
  wires:
  Demux/3 -> Mux8/1
  Demux/2 -> Mux7/1
  Demux1/1 -> Mux6/2
  Demux/1 -> Mux6/1
  Product/1 -> RB/1
  Demux/4 -> Mux9/1
  Mux6/1 -> Product/2
  Demux1/4 -> Mux9/2
  Mux7/1 -> Product1/2
  Mux9/1 -> Product3/2
  Measured/1 -> Demux1/1
  Demux2/3 -> Product2/1
  Demux1/2 -> Mux7/2
  Desired/1 -> Demux/1
  Demux2/1 -> Product/1
  Product3/1 -> LF/1
  Product1/1 -> RF/1
  Product2/1 -> LB/1
  Mux8/1 -> Product2/2
  Demux1/3 -> Mux8/2
  Enabled/1 -> Demux2/1
  Demux2/4 -> Product3/1
  Demux2/2 -> Product1/1

== system playback_data_4/Control/Subsystem/SEA Control Toggle ==
  enable : Inport
  tau_measured : Inport  Port=2
  tau_cmd : Inport  Port=3
  Abs : Abs
  Abs1 : Abs
  But Commanding a Small Torque? : simulink/Logic and Bit Operations/Compare To Constant  relop=<  const=sea_control_torque_cmd_small_threshold  OutDataTypeStr=boolean
  Logical Operator1 : Logic  AllPortsSameDT=off  OutDataTypeStr=boolean
  Logical Operator2 : Logic  Operator=NOT  AllPortsSameDT=off  OutDataTypeStr=boolean
  Logical Operator3 : Logic  AllPortsSameDT=off  OutDataTypeStr=boolean
  Logical Operator4 : Logic  AllPortsSameDT=off  OutDataTypeStr=boolean
  Measuring a Large Torque? (High Gains) : simulink/Logic and Bit Operations/Compare To Constant  relop=>=  const=loaded_unloaded_torque_threshold  OutDataTypeStr=boolean
  SEA Control on/off [1/0] : Outport
  wires:
  But Commanding a Small Torque?/1 -> Logical Operator1/2
  Logical Operator1/1 -> Logical Operator4/2
  tau_cmd/1 -> Abs/1
  Abs/1 -> But Commanding a Small Torque?/1
  tau_measured/1 -> Abs1/1
  Abs1/1 -> Measuring a Large Torque? (High Gains)/1
  Logical Operator3/1 -> SEA Control on/off [1/0]/1
  Logical Operator2/1 -> Logical Operator3/2
  Logical Operator4/1 -> Logical Operator2/1
  enable/1 -> Logical Operator4/1, Logical Operator3/1
  Measuring a Large Torque? (High Gains)/1 -> Logical Operator1/1

== system playback_data_4/Control/Subsystem/SEA Controller (Torque) ==
  phi_load [rad] x4 : Inport
  phi_gear [rad] x4 : Inport  Port=2
  tau_des sagittal [Nm] x4 : Inport  Port=3
  dtau_des sagittal [Nm] x4 : Inport  Port=4
  dphi_load [rad/s] x4 : Inport  Port=5
  dphi_gear [rad/s] x4 : Inport  Port=6
  Abs : Abs
  Antiresonance Compensation : Subsystem
  Friction Compensation : Subsystem
  Loaded Unloaded Switch : Subsystem
  P gain ramp : Lookup_n-D  NumberOfTableDimensions=1  BreakpointsForDimension1=gain_nodes_sea_torque  Table=kp_sea_torque  InternalRulePriority=Speed  RndMeth=Simplest  InputSameDT=on
  Product : Product  SampleTime=sample_time  RndMeth=Zero
  Product2 : Product  RndMeth=Zero
  Spring Stiffness : Gain  Gain=k_sea
  Spring Stiffness 1 : Gain  Gain=k_sea
  Sum1 : Sum  Inputs=-+|
  Sum10 : Sum  Inputs=|++
  Sum2 : Sum  Inputs=|+-
  Sum3 : Sum  Inputs=++|
  Sum5 : Sum  Inputs=|+-
  Sum6 : Sum  Inputs=-+|
  Sum7 : Sum  Inputs=+|+
  Torque Limiter (outside) 1 : Saturate  UpperLimit=max_sagittal_loaded_torque  LowerLimit=-max_sagittal_loaded_torque
      settings: AttributesFormatString=Hi: %<UpperLimit>\nLo: %<LowerLimit>
  Torque Limiter (outside) 3 : Saturate  UpperLimit=max_sagittal_unloaded_torque  LowerLimit=-max_sagittal_unloaded_torque
      settings: AttributesFormatString=Hi: %<UpperLimit>\nLo: %<LowerLimit>
  Torque Threshold : simulink/Logic and Bit Operations/Compare To Constant  relop=>=  const=loaded_unloaded_torque_threshold  OutDataTypeStr=boolean
  critical damping : Subsystem
  tau_cmd sagittal [Nm] x4 : Outport
  tau_measured [Nm] x4 : Outport  Port=2
  wires:
  Product2/1 -> Sum7/2
  Sum2/1 -> Product2/2
  Sum5/1 -> Product/2
  dphi_gear [rad/s] x4/1 -> Friction Compensation/1(Motor Velocity [rad/s]), Sum6/2
  dphi_load [rad/s] x4/1 -> Sum6/1
  Spring Stiffness 1/1 -> Sum2/2
  Sum6/1 -> Spring Stiffness 1/1
  dtau_des sagittal [Nm] x4/1 -> Sum2/1
  tau_des sagittal [Nm] x4/1 -> Sum5/1
  phi_gear [rad] x4/1 -> Sum1/2
  phi_load [rad] x4/1 -> Sum1/1
  Sum1/1 -> Spring Stiffness/1
  Spring Stiffness/1 -> Sum3/1, Sum5/2, Abs/1, tau_measured [Nm] x4/1
  Sum10/1 -> Antiresonance Compensation/1(Torque), Torque Limiter (outside) 1/1
  P gain ramp/1 -> critical damping/1(p gain), Product/1
  Product/1 -> Sum7/1
  Sum7/1 -> Sum3/2
  Torque Limiter (outside) 1/1 -> Loaded Unloaded Switch/1(Loaded Signal)
  Torque Limiter (outside) 3/1 -> Loaded Unloaded Switch/2(Unloaded Signal)
  Antiresonance Compensation/1(Filtered Torque) -> Torque Limiter (outside) 3/1
  Friction Compensation/1(Friction Compensation [Nm]) -> Sum10/2
  Loaded Unloaded Switch/1(Signal) -> tau_cmd sagittal [Nm] x4/1
  Torque Threshold/1 -> Loaded Unloaded Switch/3(Loaded/Unloaded [1/0] x4)
  Abs/1 -> P gain ramp/1, Torque Threshold/1
  Sum3/1 -> Sum10/1
  critical damping/1(d gain) -> Product2/1

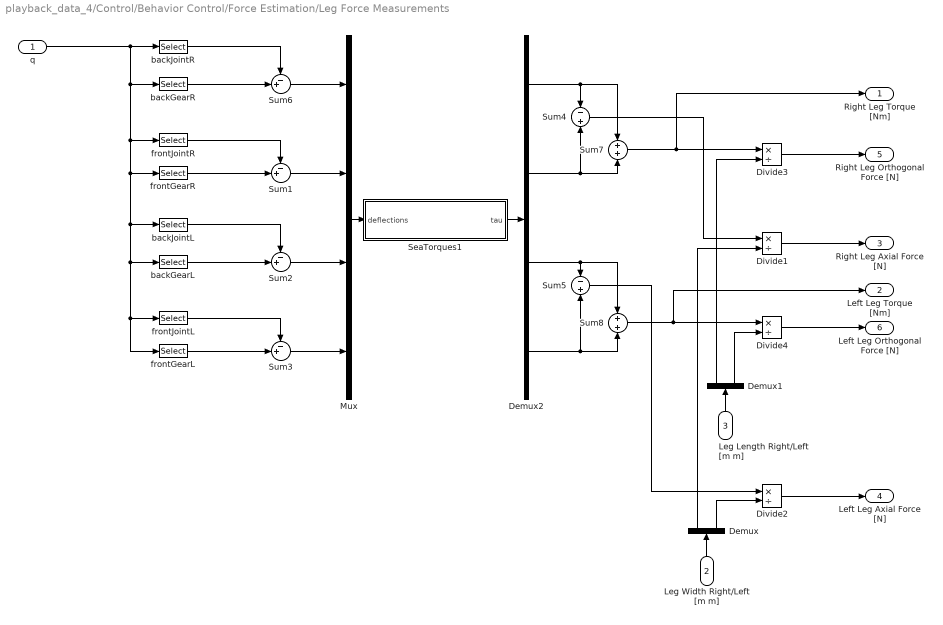
== system playback_data_4/Control/Behavior Control/Force Estimation/Leg Force Measurements ==
  q : Inport
  Leg Width Right/Left [m m] : Inport  Port=2
  Leg Length Right/Left [m m] : Inport  Port=3
  Demux : Demux  Outputs=2
  Demux1 : Demux  Outputs=2
  Demux2 : Demux
  Divide{1..4} (4 alike) : Product  Inputs=*/
  Mux : Mux
  SeaTorques1 : MATLAB Function  TreatAsAtomicUnit=on
  Sum{1..3,6} (4 alike) : Sum  Inputs=-+|
  Sum4 : Sum  Inputs=-|+
  Sum5 : Sum  Inputs=-|+
  Sum7 : Sum  Inputs=+|+
  Sum8 : Sum  Inputs=+|+
  backGearL : Selector  InputPortWidth=13  Indices=[6]
  backGearR : Selector  InputPortWidth=13  Indices=[2]
  backJointL : Selector  InputPortWidth=13  Indices=[5]
  backJointR : Selector  InputPortWidth=13  Indices=[1]
  frontGearL : Selector  InputPortWidth=13  Indices=[8]
  frontGearR : Selector  InputPortWidth=13  Indices=[4]
  frontJointL : Selector  InputPortWidth=13  Indices=[7]
  frontJointR : Selector  InputPortWidth=13  Indices=[3]
  Right Leg Torque [Nm] : Outport
  Left Leg Torque [Nm] : Outport  Port=2
  Right Leg Axial Force [N] : Outport  Port=3
  Left Leg Axial Force [N] : Outport  Port=4
  Right Leg Orthogonal Force [N] : Outport  Port=5
  Left Leg Orthogonal Force [N] : Outport  Port=6
  wires:
  SeaTorques1/1(tau) -> Demux2/1
  Mux/1 -> SeaTorques1/1(deflections)
  Divide4/1 -> Left Leg Orthogonal Force [N]/1
  Divide3/1 -> Right Leg Orthogonal Force [N]/1
  Leg Length Right/Left [m m]/1 -> Demux1/1
  Demux1/2 -> Divide4/2
  Demux1/1 -> Divide3/2
  Sum8/1 -> Left Leg Torque [Nm]/1, Divide4/1
  Sum7/1 -> Right Leg Torque [Nm]/1, Divide3/1
  Demux2/3 -> Sum5/1, Sum8/1
  Divide2/1 -> Left Leg Axial Force [N]/1
  Divide1/1 -> Right Leg Axial Force [N]/1
  Demux/2 -> Divide2/2
  Demux/1 -> Divide1/2
  Leg Width Right/Left [m m]/1 -> Demux/1
  Sum5/1 -> Divide2/1
  Sum4/1 -> Divide1/1
  Demux2/4 -> Sum8/2, Sum5/2
  Demux2/2 -> Sum4/2, Sum7/2
  Demux2/1 -> Sum7/1, Sum4/1
  q/1 -> backJointR/1, frontJointR/1, frontGearR/1, backGearL/1, frontGearL/1, frontJointL/1, backJointL/1, backGearR/1
  backGearR/1 -> Sum6/2
  frontJointR/1 -> Sum1/1
  frontGearR/1 -> Sum1/2
  backJointR/1 -> Sum6/1
  Sum1/1 -> Mux/2
  Sum6/1 -> Mux/1
  backGearL/1 -> Sum2/2
  frontJointL/1 -> Sum3/1
  frontGearL/1 -> Sum3/2
  backJointL/1 -> Sum2/1
  Sum2/1 -> Mux/3
  Sum3/1 -> Mux/4

== system playback_data_4/Control/Behavior Control/Force Estimation/Leg Plane GRF ==
  Axial Force [N] : Inport
  Orthogonal Force [N] : Inport  Port=2
  Torso Pitch [rad] : Inport  Port=3
  Leg Angle [rad] : Inport  Port=4
  Gain : Gain  Gain=-1
  Product : Product
  Product1 : Product
  Sum : Sum  Inputs=++|
  Sum1 : Sum  Inputs=+|+
  Trigonometric Function : Trigonometry  Operator=cos
  Trigonometric Function1 : Trigonometry
  Vertical Force [N] : Outport
  wires:
  Gain/1 -> Sum1/1
  Sum/1 -> Trigonometric Function1/1, Trigonometric Function/1
  Product/1 -> Gain/1
  Trigonometric Function/1 -> Product/2
  Torso Pitch [rad]/1 -> Sum/1
  Leg Angle [rad]/1 -> Sum/2
  Axial Force [N]/1 -> Product/1
  Orthogonal Force [N]/1 -> Product1/1
  Trigonometric Function1/1 -> Product1/2
  Sum1/1 -> Vertical Force [N]/1
  Product1/1 -> Sum1/2

== system playback_data_4/Control/Behavior Control/Primary and Lateral Behavior/Circular Buffer ==
  Flight [1/0] : Inport
  Exiting Stance [1/0] : Inport  Port=2
  Hopping [1/0] : Inport  Port=3
  dX [m/s] : Inport  Port=4
  dY [m/s] : Inport  Port=5
  X Foot Correction [m] : Inport  Port=6
  Y Foot Correction [m] : Inport  Port=7
  target dX [m/s] : Inport  Port=8
  target dY [m/s] : Inport  Port=9
  Buffer : MATLAB Function  TreatAsAtomicUnit=on  SystemSampleTime=0.001
  Buffer1 : MATLAB Function  TreatAsAtomicUnit=on  SystemSampleTime=0.001
  Buffer2 : MATLAB Function  TreatAsAtomicUnit=on  SystemSampleTime=0.001
  Buffer3 : MATLAB Function  TreatAsAtomicUnit=on  SystemSampleTime=0.001
  Buffer4 : MATLAB Function  TreatAsAtomicUnit=on  SystemSampleTime=0.001
  Buffer5 : MATLAB Function  TreatAsAtomicUnit=on  SystemSampleTime=0.001
  Buffer6 : MATLAB Function  TreatAsAtomicUnit=on  SystemSampleTime=0.001
  Buffer7 : MATLAB Function  TreatAsAtomicUnit=on  SystemSampleTime=0.001
  Demux : Demux  Outputs=6
  Detect Decrease : simulink/Logic and Bit Operations/Detect Decrease  vinit=0.0  InputProcessing=Inherited  OutDataTypeStr=boolean
  Enabled on Touchdown : Subsystem  TreatAsAtomicUnit=on
  Logical Operator : Logic  AllPortsSameDT=off  OutDataTypeStr=boolean
  Mux : Mux  Inputs=6
  buffer size5 : Constant  Value=recorded_steps
  "dX Touchdown History " : Outport
  X Foot Correction History : Outport  Port=2
  dX Takeoff History : Outport  Port=3
  "dY Touchdown History " : Outport  Port=4
  Y Foot Correction History : Outport  Port=5
  dY Takeoff History : Outport  Port=6
  target dX History : Outport  Port=7
  target dY History : Outport  Port=8
  wires:
  Buffer/1(buffer) -> "dX Touchdown History "/1
  Detect Decrease/1 -> Enabled on Touchdown/Enable
  Buffer1/1(buffer) -> X Foot Correction History/1
  Buffer2/1(buffer) -> dX Takeoff History/1
  Demux/1 -> Buffer/1(data)
  Demux/3 -> Buffer1/1(data)
  X Foot Correction [m]/1 -> Mux/3
  Buffer3/1(buffer) -> "dY Touchdown History "/1
  Buffer4/1(buffer) -> Y Foot Correction History/1
  Demux/2 -> Buffer3/1(data)
  Buffer5/1(buffer) -> dY Takeoff History/1
  Y Foot Correction [m]/1 -> Mux/4
  Demux/4 -> Buffer4/1(data)
  target dX [m/s]/1 -> Mux/5
  Buffer6/1(buffer) -> target dX History/1
  Buffer7/1(buffer) -> target dY History/1
  buffer size5/1 -> Buffer2/3(buffer_size), Buffer/3(buffer_size), Buffer7/3(buffer_size), Buffer6/3(buffer_size), Buffer4/3(buffer_size), Buffer1/3(buffer_size), Buffer3/3(buffer_size), Buffer5/3(buffer_size)
  Demux/6 -> Buffer7/1(data)
  Demux/5 -> Buffer6/1(data)
  target dY [m/s]/1 -> Mux/6
  Exiting Stance [1/0]/1 -> Buffer/2(trigger), Buffer7/2(trigger), Buffer6/2(trigger), Buffer4/2(trigger), Buffer1/2(trigger), Buffer3/2(trigger), Buffer2/2(trigger), Buffer5/2(trigger)
  Hopping [1/0]/1 -> Logical Operator/1
  dY [m/s]/1 -> Buffer5/1(data), Mux/2
  dX [m/s]/1 -> Buffer2/1(data), Mux/1
  Flight [1/0]/1 -> Logical Operator/2
  Logical Operator/1 -> Detect Decrease/1
  Mux/1 -> Enabled on Touchdown/1(In)
  Enabled on Touchdown/1(Out) -> Demux/1

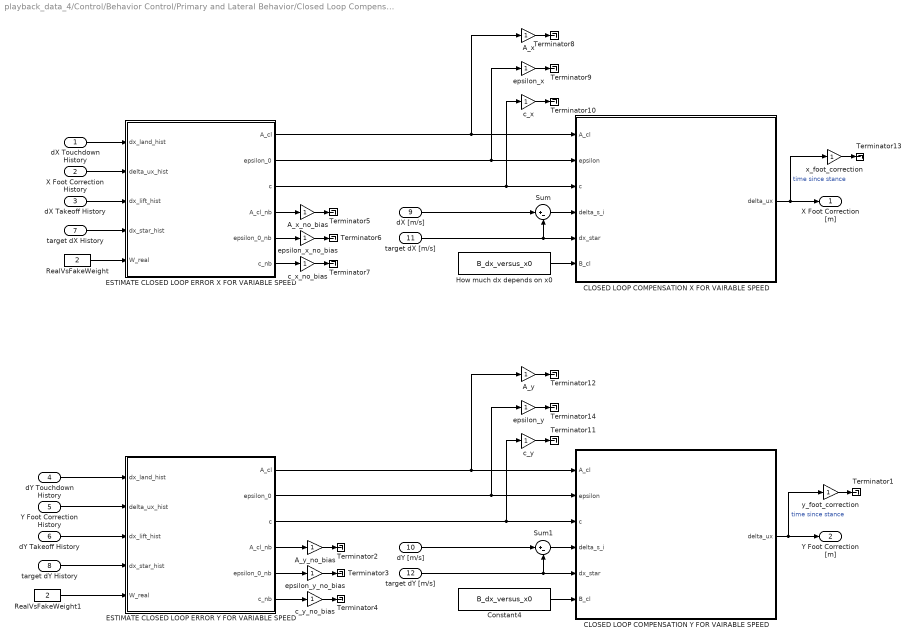
== system playback_data_4/Control/Behavior Control/Primary and Lateral Behavior/Closed Loop Compensation ==
  dX Touchdown History : Inport
  X Foot Correction History : Inport  Port=2
  dX Takeoff History : Inport  Port=3
  dY Touchdown History : Inport  Port=4
  Y Foot Correction History : Inport  Port=5
  dY Takeoff History : Inport  Port=6
  target dX History : Inport  Port=7
  target dY History : Inport  Port=8
  dX [m/s] : Inport  Port=9
  dY [m/s] : Inport  Port=10
  target dX [m/s] : Inport  Port=11
  "target dY [m/s] " : Inport  Port=12
  A_x : Gain
  A_x_no_bias : Gain
  A_y : Gain
  A_y_no_bias : Gain
  CLOSED LOOP COMPENSATION X FOR VAIRABLE SPEED : MATLAB Function  TreatAsAtomicUnit=on
  CLOSED LOOP COMPENSATION Y FOR VAIRABLE SPEED : MATLAB Function  TreatAsAtomicUnit=on
  Constant4 : Constant  Value=B_dx_versus_x0
  ESTIMATE CLOSED LOOP ERROR X FOR VARIABLE SPEED : MATLAB Function  TreatAsAtomicUnit=on
  ESTIMATE CLOSED LOOP ERROR Y FOR VARIABLE SPEED : MATLAB Function  TreatAsAtomicUnit=on
  How much dx depends on x0 : Constant  Value=B_dx_versus_x0
  RealVsFakeWeight : Constant  Value=2
  RealVsFakeWeight1 : Constant  Value=2
  Sum : Sum  Inputs=|+-
  Sum1 : Sum  Inputs=|+-
  Terminator{1..14} (14 alike) : Terminator
  c_x : Gain
  c_x_no_bias : Gain
  c_y : Gain
  c_y_no_bias : Gain
  epsilon_x : Gain
  epsilon_x_no_bias : Gain
  epsilon_y : Gain
  epsilon_y_no_bias : Gain
  x_foot_correction : Gain
  y_foot_correction : Gain
  X Foot Correction [m] : Outport
  Y Foot Correction [m] : Outport  Port=2
  wires:
  c_y/1 -> Terminator11/1
  epsilon_y/1 -> Terminator14/1
  A_y/1 -> Terminator12/1
  ESTIMATE CLOSED LOOP ERROR Y FOR VARIABLE SPEED/1(A_cl) -> CLOSED LOOP COMPENSATION Y FOR VAIRABLE SPEED/1(A_cl), A_y/1
  ESTIMATE CLOSED LOOP ERROR Y FOR VARIABLE SPEED/2(epsilon_0) -> CLOSED LOOP COMPENSATION Y FOR VAIRABLE SPEED/2(epsilon), epsilon_y/1
  ESTIMATE CLOSED LOOP ERROR Y FOR VARIABLE SPEED/3(c) -> CLOSED LOOP COMPENSATION Y FOR VAIRABLE SPEED/3(c), c_y/1
  c_x/1 -> Terminator10/1
  epsilon_x/1 -> Terminator9/1
  A_x/1 -> Terminator8/1
  ESTIMATE CLOSED LOOP ERROR X FOR VARIABLE SPEED/1(A_cl) -> CLOSED LOOP COMPENSATION X FOR VAIRABLE SPEED/1(A_cl), A_x/1
  ESTIMATE CLOSED LOOP ERROR X FOR VARIABLE SPEED/2(epsilon_0) -> CLOSED LOOP COMPENSATION X FOR VAIRABLE SPEED/2(epsilon), epsilon_x/1
  ESTIMATE CLOSED LOOP ERROR X FOR VARIABLE SPEED/3(c) -> CLOSED LOOP COMPENSATION X FOR VAIRABLE SPEED/3(c), c_x/1
  ESTIMATE CLOSED LOOP ERROR Y FOR VARIABLE SPEED/6(c_nb) -> c_y_no_bias/1
  ESTIMATE CLOSED LOOP ERROR Y FOR VARIABLE SPEED/5(epsilon_0_nb) -> epsilon_y_no_bias/1
  ESTIMATE CLOSED LOOP ERROR Y FOR VARIABLE SPEED/4(A_cl_nb) -> A_y_no_bias/1
  c_y_no_bias/1 -> Terminator4/1
  epsilon_y_no_bias/1 -> Terminator3/1
  A_y_no_bias/1 -> Terminator2/1
  c_x_no_bias/1 -> Terminator7/1
  epsilon_x_no_bias/1 -> Terminator6/1
  A_x_no_bias/1 -> Terminator5/1
  ESTIMATE CLOSED LOOP ERROR X FOR VARIABLE SPEED/4(A_cl_nb) -> A_x_no_bias/1
  ESTIMATE CLOSED LOOP ERROR X FOR VARIABLE SPEED/5(epsilon_0_nb) -> epsilon_x_no_bias/1
  ESTIMATE CLOSED LOOP ERROR X FOR VARIABLE SPEED/6(c_nb) -> c_x_no_bias/1
  y_foot_correction/1 -> Terminator1/1
  CLOSED LOOP COMPENSATION Y FOR VAIRABLE SPEED/1(delta_ux) -> Y Foot Correction [m]/1, y_foot_correction/1  "time since stance"
  x_foot_correction/1 -> Terminator13/1
  CLOSED LOOP COMPENSATION X FOR VAIRABLE SPEED/1(delta_ux) -> X Foot Correction [m]/1, x_foot_correction/1  "time since stance"
  Sum1/1 -> CLOSED LOOP COMPENSATION Y FOR VAIRABLE SPEED/4(delta_s_i)
  dY Touchdown History/1 -> ESTIMATE CLOSED LOOP ERROR Y FOR VARIABLE SPEED/1(dx_land_hist)
  dX [m/s]/1 -> Sum/1
  dX Touchdown History/1 -> ESTIMATE CLOSED LOOP ERROR X FOR VARIABLE SPEED/1(dx_land_hist)
  dX Takeoff History/1 -> ESTIMATE CLOSED LOOP ERROR X FOR VARIABLE SPEED/3(dx_lift_hist)
  X Foot Correction History/1 -> ESTIMATE CLOSED LOOP ERROR X FOR VARIABLE SPEED/2(delta_ux_hist)
  target dX History/1 -> ESTIMATE CLOSED LOOP ERROR X FOR VARIABLE SPEED/4(dx_star_hist)
  target dX [m/s]/1 -> CLOSED LOOP COMPENSATION X FOR VAIRABLE SPEED/5(dx_star), Sum/2
  Sum/1 -> CLOSED LOOP COMPENSATION X FOR VAIRABLE SPEED/4(delta_s_i)
  How much dx depends on x0/1 -> CLOSED LOOP COMPENSATION X FOR VAIRABLE SPEED/6(B_cl)
  RealVsFakeWeight/1 -> ESTIMATE CLOSED LOOP ERROR X FOR VARIABLE SPEED/5(W_real)
  dY [m/s]/1 -> Sum1/1
  dY Takeoff History/1 -> ESTIMATE CLOSED LOOP ERROR Y FOR VARIABLE SPEED/3(dx_lift_hist)
  Y Foot Correction History/1 -> ESTIMATE CLOSED LOOP ERROR Y FOR VARIABLE SPEED/2(delta_ux_hist)
  target dY History/1 -> ESTIMATE CLOSED LOOP ERROR Y FOR VARIABLE SPEED/4(dx_star_hist)
  "target dY [m/s] "/1 -> CLOSED LOOP COMPENSATION Y FOR VAIRABLE SPEED/5(dx_star), Sum1/2
  Constant4/1 -> CLOSED LOOP COMPENSATION Y FOR VAIRABLE SPEED/6(B_cl)
  RealVsFakeWeight1/1 -> ESTIMATE CLOSED LOOP ERROR Y FOR VARIABLE SPEED/5(W_real)

== system playback_data_4/Control/Behavior Control/Primary and Lateral Behavior/Enabled on Takeoff ==
  In : Inport
  Enable : EnablePort
  Out : Outport
  wires:
  In/1 -> Out/1
